simulink model "aircraft_pitch_multibody"  (R2022b)
settings: Solver=ode23t  StartTime=0.0  StopTime=stopTime  MaxStep=0.005  RelTol=1e-9  AbsTol=1e-11
model workspace (MAT data in the model file):
  Jpitch = 1
  Kd = 2.98
  Ki = 1.74
  Kp = 5.1852
  N = 100
  aScale = 1
  antiWindup = 0
  biasAcceleration = 0
  biasTime = 20
  deltaMax = inf
  geometryInertia = 4.77572166667
  massScale = 1
  r = 0.2
  stopTime = 100
undefined symbols (not defined in the file or in its folder): X, Y, Z
libraries: sm_lib x9, nesl_utility x4
settings Model: Creator=shark  LastModifiedBy=shark

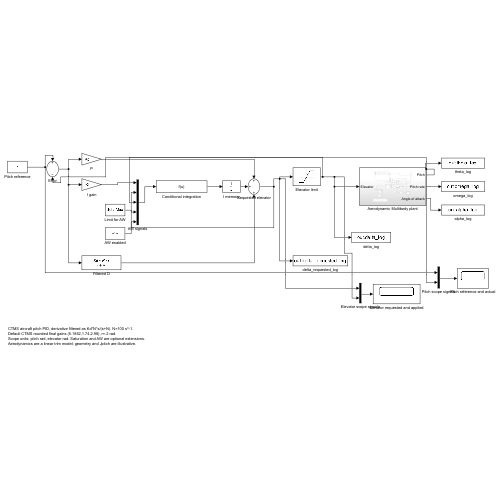
[thumbnail: Simulink's stored preview of the top-level diagram]
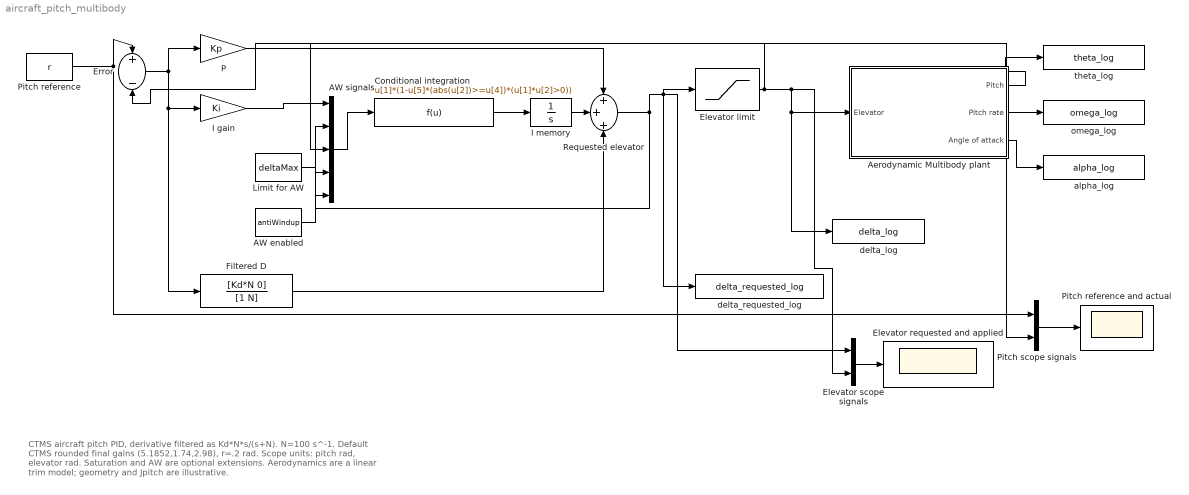
== system aircraft_pitch_multibody ==
  note: CTMS aircraft pitch PID, derivative filtered as Kd*N*s/(s+N). N=100 s^-1.
      | Default CTMS rounded final gains (5.1852,1.74,2.98), r=.2 rad.
      | Scope units: pitch rad, elevator rad. Saturation and AW are optional extensions.
      | Aerodynamics are a linear trim model; geometry and Jpitch are illustrative.
  AW enabled : Constant  Value=antiWindup
  AW signals : Mux  Inputs=5
  Aerodynamic Multibody plant : Subsystem
  Conditional integration : Fcn  Expr=u[1]*(1-u[5]*(abs(u[2])>=u[4])*(u[1]*u[2]>0))
  Elevator limit : Saturate  UpperLimit=deltaMax  LowerLimit=-deltaMax
  Elevator requested and applied : Scope
  Elevator scope signals : Mux  Inputs=2
  Error : Sum  Inputs=+-
  Filtered D : TransferFcn  Numerator=[Kd*N 0]  Denominator=[1 N]
  I gain : Gain  Gain=Ki
  I memory : Integrator
  Limit for AW : Constant  Value=deltaMax
  P : Gain  Gain=Kp
  Pitch reference : Constant  Value=r
  Pitch reference and actual : Scope
  Pitch scope signals : Mux  Inputs=2
  Requested elevator : Sum  Inputs=+++
  alpha_log : ToWorkspace  VariableName=alpha_log  SaveFormat=Timeseries  SampleTime=-1
  delta_log : ToWorkspace  VariableName=delta_log  SaveFormat=Timeseries  SampleTime=-1
  delta_requested_log : ToWorkspace  VariableName=delta_requested_log  SaveFormat=Timeseries  SampleTime=-1
  omega_log : ToWorkspace  VariableName=omega_log  SaveFormat=Timeseries  SampleTime=-1
  theta_log : ToWorkspace  VariableName=theta_log  SaveFormat=Timeseries  SampleTime=-1
  wires:
  Pitch reference/1 -> Error/1, Pitch scope signals/1
  Aerodynamic Multibody plant/1(Pitch) -> theta_log/1, Error/2, Pitch scope signals/2
  Error/1 -> I gain/1, Filtered D/1, P/1
  I gain/1 -> AW signals/1
  Requested elevator/1 -> AW signals/2, Elevator limit/1, delta_requested_log/1, Elevator scope signals/1
  Elevator limit/1 -> Aerodynamic Multibody plant/1(Elevator), delta_log/1, Elevator scope signals/2, AW signals/3
  Limit for AW/1 -> AW signals/4
  AW enabled/1 -> AW signals/5
  AW signals/1 -> Conditional integration/1
  Conditional integration/1 -> I memory/1
  P/1 -> Requested elevator/1
  I memory/1 -> Requested elevator/2
  Filtered D/1 -> Requested elevator/3
  Aerodynamic Multibody plant/2(Pitch rate) -> omega_log/1
  Aerodynamic Multibody plant/3(Angle of attack) -> alpha_log/1
  Pitch scope signals/1 -> Pitch reference and actual/1
  Elevator scope signals/1 -> Elevator requested and applied/1

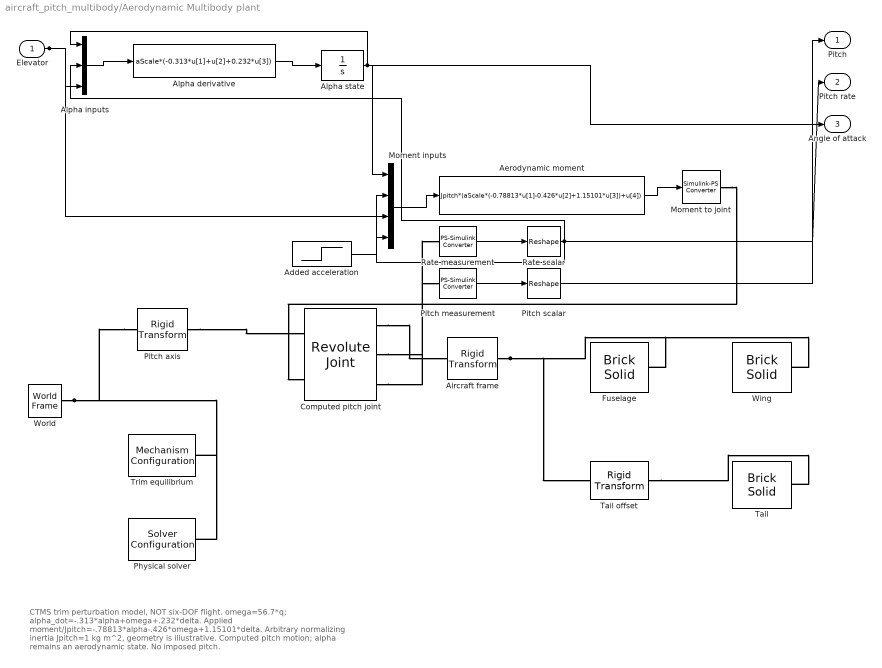
== system aircraft_pitch_multibody/Aerodynamic Multibody plant ==
  note: CTMS trim perturbation model, NOT six-DOF flight.
      | omega=56.7*q; alpha_dot=-.313*alpha+omega+.232*delta.
      | Applied moment/Jpitch=-.78813*alpha-.426*omega+1.15101*delta.
      | Arbitrary normalizing inertia Jpitch=1 kg m^2, geometry is illustrative.
      | Computed pitch motion; alpha remains an aerodynamic state. No imposed pitch.
  Elevator : Inport
  Added acceleration : Step  Time=biasTime  After=biasAcceleration  SampleTime=0
  Aerodynamic moment : Fcn  Expr=Jpitch*(aScale*(-0.78813*u[1]-0.426*u[2]+1.15101*u[3])+u[4])
  Aircraft frame : sm_lib/Frames and Transforms/Rigid Transform  TranslationMethod=None  TranslationStandardOffset=0  TranslationLengthUnit=m  TranslationStandardAxis=+Z  TranslationCartesianOffset=[0 0 0]  TranslationROffset=0  TranslationROffsetUnits=m  TranslationZOffset=0  TranslationZOffsetUnits=m  TranslationThetaOffset=0  TranslationThetaOffsetUnits=deg  RotationMethod=StandardAxis  RotationAngleUnits=deg  RotationStandardAxis=+X  RotationAngle=-90  RotationArbitraryAxis=[0 0 1]  FollAlignAxisA=+X  BaseAlignAxisA=+Y  FollAlignAxisB=+Y  BaseAlignAxisB=+Z  RotationSequenceAxes=FollowerAxes  RotationSequence=XYX  RotationSequenceAngles=[0 0 0]  RotationSequenceAnglesUnits=deg  RotationMatrix=[1 0 0; 0 1 0; 0 0 1]  Quaternion=[1 0 0 0]
  Alpha derivative : Fcn  Expr=aScale*(-0.313*u[1]+u[2]+0.232*u[3])
  Alpha inputs : Mux  Inputs=3
  Alpha state : Integrator
  Computed pitch joint : sm_lib/Joints/Revolute Joint  JointMode=Normal  SenseConstraintForce=off  SenseConstraintForceX=off  SenseConstraintForceY=off  SenseConstraintForceZ=off  SenseConstraintTorque=off  SenseConstraintTorqueX=off  SenseConstraintTorqueY=off  SenseConstraintTorqueZ=off  SenseTotalForce=off  SenseTotalForceX=off  SenseTotalForceY=off  SenseTotalForceZ=off  SenseTotalTorque=off  SenseTotalTorqueX=off  SenseTotalTorqueY=off  SenseTotalTorqueZ=off  CompositeWrenchDir=FollowerOnBase  CompositeWrenchFrame=BaseFrame  EquilibriumPosition=0  EquilibriumPositionUnits=deg  SpringStiffness=0  SpringStiffnessUnits=N*m/deg  DampingCoefficient=0  DampingCoefficientUnits=N*m/(deg/s)  TorqueActuationMode=InputTorque  MotionActuationMode=ComputedMotion  SensePosition=on  SenseVelocity=on  SenseAcceleration=off  SenseTorqueForce=off  SenseLowerLimitTorqueForce=off  SenseUpperLimitTorqueForce=off  LowerLimitSpecify=off  LowerLimitBound=-90  LowerLimitBoundUnits=deg  LowerLimitStiffness=1e4  LowerLimitStiffnessUnits=N*m/deg  LowerLimitDamping=10  LowerLimitDampingUnits=N*m/(deg/s)  LowerLimitTransitionRegionWidth=0.1  LowerLimitTransitionRegionWidthUnits=deg  UpperLimitSpecify=off  UpperLimitBound=90  UpperLimitBoundUnits=deg  UpperLimitStiffness=1e4  UpperLimitStiffnessUnits=N*m/deg  UpperLimitDamping=10  UpperLimitDampingUnits=N*m/(deg/s)  UpperLimitTransitionRegionWidth=0.1  UpperLimitTransitionRegionWidthUnits=deg  PositionTargetSpecify=on  PositionTargetPriority=High  PositionTargetValue=0  PositionTargetValueUnits=rad  VelocityTargetSpecify=on  VelocityTargetPriority=High  VelocityTargetValue=0  VelocityTargetValueUnits=rad/s
  Fuselage : sm_lib/Body Elements/Brick Solid  GraphicAmbientColor=[0.15 0.15 0.15 1.0]  BasedOnType=Mass  BrickDimensions=[8 .65 .65]  BrickDimensionUnits=m  CenterOfMass=[0 0 0]  CenterOfMassUnits=m  GraphicDiffuseColor=[.15 .45 .85]  Density=1000  DensityUnits=kg/m^3  DoExposeReferenceFrame=on  GraphicEmissiveColor=[0.0 0.0 0.0 1.0]  ExportEntireGeometry=off  SerializedFrames=<Frames/>  MarkerShape=Sphere  MarkerSize=10  GraphicType=FromGeometry  InertiaType=CalculateFromGeometry  Mass=.8*Jpitch/geometryInertia  MassUnits=kg  MomentsOfInertia=[1 1 1]  MomentsOfInertiaUnits=kg*m^2  GraphicOpacity=1.0  ProductsOfInertia=[0 0 0]  ProductsOfInertiaUnits=kg*m^2  GraphicShininess=75  GraphicSpecularColor=[0.5 0.5 0.5 1.0]  GraphicVisPropType=SimpleVisualProperties
  Moment inputs : Mux
  Moment to joint : nesl_utility/Simulink-PS Converter  PhysicalDomain=network_engine_domain  SubClassName=ps_input  LeftPortType=input  RightPortType=output  PseudoPeriodic=off  Frequencies=[]  NoiseDistribution=none  NoiseParameters=[]  Unit=N*m  AffineConversion=off  FilteringAndDerivatives=provide  SimscapeFilterOrder=1  InputFilterTimeConstant=0.001  UdotUserProvided=0
  Physical solver : nesl_utility/Solver Configuration  PhysicalDomain=network_engine_domain  SubClassName=solver  LeftPortType=input  RightPortType=generic  Tones=[]  Harmonics=[]  SimulateNoise=off  Profile=off  UseLocalSampling=off  EnableSwitchedLinearOptims=on  FrequencyDomain=off  UseCCode=off  RelTol=0.001  AbsTol=0.001  MinStep=1e-09  ToWorkspace=off  RevertToSquareIcSolve=off  NumHomotopyIterations=100  PhasorMode=off  PhasorModeNumHarmonics=1  ConsistencySolver=NEWTON_XTOL_AFTER_FTOL  IndexReductionMethod=DerivativeReplacement  DoDC=off  ResidualTolerance=1e-09  ConsistencyTolSource=GLOBAL  ConsistencyAbsTol=0.001  ConsistencyRelTol=0.001  ConsistencyTolFactor=0.001  UseLocalSolver=off  LocalSolverChoice=NE_BACKWARD_EULER_ADVANCER  ResolveIndetEquations=on  FunctionEvalNumThread=1  LocalSolverSampleTime=0.001  DoFixedCost=off  MaxNonlinIter=3  MaxModeIter=2  ComputeImpulses=off  ImpulseIterations=2  LinearAlgebra=auto  LinearAlgebraNumThread=0  EquationFormulation=NE_TIME_EF  DelaysMemoryBudget=1024  AutomaticFiltering=on  FilteringTimeConstant=0.001  PartitionStorageMethod=AS_NEEDED  PartitionMemoryBudget=1024  PartitionMethod=ROBUST
  Pitch axis : sm_lib/Frames and Transforms/Rigid Transform  TranslationMethod=None  TranslationStandardOffset=0  TranslationLengthUnit=m  TranslationStandardAxis=+Z  TranslationCartesianOffset=[0 0 0]  TranslationROffset=0  TranslationROffsetUnits=m  TranslationZOffset=0  TranslationZOffsetUnits=m  TranslationThetaOffset=0  TranslationThetaOffsetUnits=deg  RotationMethod=StandardAxis  RotationAngleUnits=deg  RotationStandardAxis=+X  RotationAngle=90  RotationArbitraryAxis=[0 0 1]  FollAlignAxisA=+X  BaseAlignAxisA=+Y  FollAlignAxisB=+Y  BaseAlignAxisB=+Z  RotationSequenceAxes=FollowerAxes  RotationSequence=XYX  RotationSequenceAngles=[0 0 0]  RotationSequenceAnglesUnits=deg  RotationMatrix=[1 0 0; 0 1 0; 0 0 1]  Quaternion=[1 0 0 0]
  Pitch measurement : nesl_utility/PS-Simulink Converter  PhysicalDomain=network_engine_domain  SubClassName=ps_output  LeftPortType=input  RightPortType=output  PseudoPeriodic=off  Frequencies=[]  VectorFormat=inherit  Unit=rad  AffineConversion=off
  Pitch scalar : Reshape
  Rate measurement : nesl_utility/PS-Simulink Converter  PhysicalDomain=network_engine_domain  SubClassName=ps_output  LeftPortType=input  RightPortType=output  PseudoPeriodic=off  Frequencies=[]  VectorFormat=inherit  Unit=rad/s  AffineConversion=off
  Rate scalar : Reshape
  Tail : sm_lib/Body Elements/Brick Solid  GraphicAmbientColor=[0.15 0.15 0.15 1.0]  BasedOnType=Mass  BrickDimensions=[1 3 .1]  BrickDimensionUnits=m  CenterOfMass=[0 0 0]  CenterOfMassUnits=m  GraphicDiffuseColor=[.3 .55 .85]  Density=1000  DensityUnits=kg/m^3  DoExposeReferenceFrame=on  GraphicEmissiveColor=[0.0 0.0 0.0 1.0]  ExportEntireGeometry=off  SerializedFrames=<Frames/>  MarkerShape=Sphere  MarkerSize=10  GraphicType=FromGeometry  InertiaType=CalculateFromGeometry  Mass=.05*Jpitch/geometryInertia  MassUnits=kg  MomentsOfInertia=[1 1 1]  MomentsOfInertiaUnits=kg*m^2  GraphicOpacity=1.0  ProductsOfInertia=[0 0 0]  ProductsOfInertiaUnits=kg*m^2  GraphicShininess=75  GraphicSpecularColor=[0.5 0.5 0.5 1.0]  GraphicVisPropType=SimpleVisualProperties
  Tail offset : sm_lib/Frames and Transforms/Rigid Transform  TranslationMethod=Cartesian  TranslationStandardOffset=0  TranslationLengthUnit=m  TranslationStandardAxis=+Z  TranslationCartesianOffset=[-3 0 .2]  TranslationROffset=0  TranslationROffsetUnits=m  TranslationZOffset=0  TranslationZOffsetUnits=m  TranslationThetaOffset=0  TranslationThetaOffsetUnits=deg  RotationMethod=None  RotationAngleUnits=deg  RotationStandardAxis=+Z  RotationAngle=0.0  RotationArbitraryAxis=[0 0 1]  FollAlignAxisA=+X  BaseAlignAxisA=+Y  FollAlignAxisB=+Y  BaseAlignAxisB=+Z  RotationSequenceAxes=FollowerAxes  RotationSequence=XYX  RotationSequenceAngles=[0 0 0]  RotationSequenceAnglesUnits=deg  RotationMatrix=[1 0 0; 0 1 0; 0 0 1]  Quaternion=[1 0 0 0]
  Trim equilibrium : sm_lib/Utilities/Mechanism Configuration  UniformGravity=Constant  GravityVector=[0 0 0]  GravityUnits=m/s^2  LinearizationDelta=0.001  JointModeTransitionNonlinearIterations=2
  Wing : sm_lib/Body Elements/Brick Solid  GraphicAmbientColor=[0.15 0.15 0.15 1.0]  BasedOnType=Mass  BrickDimensions=[1.4 8 .12]  BrickDimensionUnits=m  CenterOfMass=[0 0 0]  CenterOfMassUnits=m  GraphicDiffuseColor=[.65 .75 .9]  Density=1000  DensityUnits=kg/m^3  DoExposeReferenceFrame=on  GraphicEmissiveColor=[0.0 0.0 0.0 1.0]  ExportEntireGeometry=off  SerializedFrames=<Frames/>  MarkerShape=Sphere  MarkerSize=10  GraphicType=FromGeometry  InertiaType=CalculateFromGeometry  Mass=.15*Jpitch/geometryInertia  MassUnits=kg  MomentsOfInertia=[1 1 1]  MomentsOfInertiaUnits=kg*m^2  GraphicOpacity=1.0  ProductsOfInertia=[0 0 0]  ProductsOfInertiaUnits=kg*m^2  GraphicShininess=75  GraphicSpecularColor=[0.5 0.5 0.5 1.0]  GraphicVisPropType=SimpleVisualProperties
  World : sm_lib/Frames and Transforms/World Frame
  Pitch : Outport
  Pitch rate : Outport  Port=2
  Angle of attack : Outport  Port=3
  wires:
  Alpha state/1 -> Alpha inputs/1, Moment inputs/1, Angle of attack/1
  Rate scalar/1 -> Alpha inputs/2, Moment inputs/2, Pitch rate/1
  Elevator/1 -> Alpha inputs/3, Moment inputs/3
  Alpha inputs/1 -> Alpha derivative/1
  Alpha derivative/1 -> Alpha state/1
  Added acceleration/1 -> Moment inputs/4
  Moment inputs/1 -> Aerodynamic moment/1
  Aerodynamic moment/1 -> Moment to joint/1
  Pitch measurement/1 -> Pitch scalar/1
  Rate measurement/1 -> Rate scalar/1
  Pitch scalar/1 -> Pitch/1
  connections:
  Pitch axis/LConn1 -- World/RConn1 -- Trim equilibrium/RConn1 -- Physical solver/RConn1
  Pitch axis/RConn1 -- Computed pitch joint/LConn1
  Moment to joint/RConn1 -- Computed pitch joint/LConn2
  Computed pitch joint/RConn1 -- Aircraft frame/LConn1
  Computed pitch joint/RConn2 -- Pitch measurement/LConn1
  Computed pitch joint/RConn3 -- Rate measurement/LConn1
  Fuselage/RConn1 -- Aircraft frame/RConn1 -- Wing/RConn1 -- Tail offset/LConn1
  Tail offset/RConn1 -- Tail/RConn1
